simulink model "SimulinkModel"  (R2023b)
settings: Solver=FixedStepAuto  StartTime=0.0  StopTime=10.0  FixedStep=param.rateTransition_Main  RelTol=1e-3  EnableMultiTasking=on
undefined symbols (not defined in the file or in its folder): lidarMeasurement, param, SensorDataOS2, timestamp
libraries: simulink x30, GenericTarget x11, etargetslib x8
(part 2 of 3)

== system SimulinkModel/Send Dynamic Mapping/staticVoxelOccupancyColors ==
  note: uint8 	0x53 bzw 'S'
      | double 	Timestamp
      | uint8  	MaxSegment
      | uint8 	SegmentImdex
      | double 	North East Down Roll Pitch Yaw
      | uint32	FrameID
      | uint32 	num Points
      | uint32	Points : XYZ
      | total 67 bytes
  timestamp : Inport
  pose : Inport  Port=2
  point : Inport  Port=3
  numpoint : Inport  Port=4
  nummsg : Inport  Port=5
  frameID : Inport  Port=6
  Byte Pack1 : etargetslib/Byte Pack  datatypes={'uint8','double','uint8', 'uint8', 'double', 'uint32', 'uint32', 'single'}  byteAlign=1
  Cast To Double1 : DataTypeConversion  OutDataTypeStr=uint8  SaturateOnIntegerOverflow=off  RndMeth=Floor
  Cast To Double2 : DataTypeConversion  OutDataTypeStr=uint8  SaturateOnIntegerOverflow=off  RndMeth=Floor
  Constant1 : Constant  Value=-1  OutDataTypeStr=int32
  Constant2 : Constant  Value=[0x53]  OutDataTypeStr=uint8
  Constant3 : Constant  Value=[0,0,0,0]  OutDataTypeStr=uint8
  Constant4 : Constant  Value=43  OutDataTypeStr=uint32
  Constant5 : Constant  Value=115  OutDataTypeStr=uint32
  Constant6 : Constant  Value=-1  OutDataTypeStr=int32
  Constant7 : Constant  Value=1111  OutDataTypeStr=uint16
  Equal1 : RelationalOperator  Operator===  OutDataTypeStr=boolean  RndMeth=Simplest  InputSameDT=off
  For Iterator : ForIterator  ResetStates=reset  IterationSource=external
  Gain : Gain  Gain=115  OutDataTypeStr=int32
  Gain1 : Gain  Gain=12  OutDataTypeStr=uint32  LockScale=on
  Selector : Selector  NumberOfDimensions=2  IndexMode=Zero-based  InputPortWidth=3  IndexOptions=Select all,Starting index (port)  Indices=[1 3],1  OutputSizes=4e3,115
  Sum : Sum  Inputs=|++
  Sum1 : Sum  Inputs=|++  OutDataTypeStr=uint32
  Sum2 : Sum  Inputs=|++
  Sum3 : Sum  Inputs=|+-
  Switch : Switch  Criteria=u2 > Threshold  SaturateOnIntegerOverflow=off  InputSameDT=off
  UDP Send : GenericTarget/Interface/UDP Send  showDetails=off  interfacePort=1111  interfaceIP=[0,0,0,0]  deviceName=''  prioritySocket=6  allowBroadcast=off  SampleTime=-1
      settings: SourceProductName=Generic Target
  wires:
  Constant2/1 -> Byte Pack1/1
  timestamp/1 -> Byte Pack1/2
  Constant1/1 -> Sum/1
  For Iterator/1 -> Equal1/2, Sum/2
  Sum/1 -> Cast To Double2/1, Gain/1
  numpoint/1 -> Sum3/1
  Gain/1 -> Sum3/2, Selector/2
  point/1 -> Selector/1
  nummsg/1 -> Sum2/1, Equal1/1, For Iterator/1
  Equal1/1 -> Switch/2
  Sum3/1 -> Switch/1
  Constant5/1 -> Switch/3
  Selector/1 -> Byte Pack1/8
  Switch/1 -> Gain1/1, Byte Pack1/7
  frameID/1 -> Byte Pack1/6
  pose/1 -> Byte Pack1/5
  Cast To Double2/1 -> Byte Pack1/4
  Cast To Double1/1 -> Byte Pack1/3
  Sum2/1 -> Cast To Double1/1
  Constant6/1 -> Sum2/2
  Constant4/1 -> Sum1/1
  Gain1/1 -> Sum1/2
  Sum1/1 -> UDP Send/4
  Byte Pack1/1 -> UDP Send/3
  Constant7/1 -> UDP Send/2
  Constant3/1 -> UDP Send/1

== system SimulinkModel/Send Dynamic Mapping/staticVoxelReflectivityColors ==
  note: uint8 	0x53 bzw 'S'
      | double 	Timestamp
      | uint8  	MaxSegment
      | uint8 	SegmentImdex
      | double 	North East Down
      | uint32	FrameID
      | uint32 	num Points
      | uint32	Points : XYZ
      | total 43 bytes
  timestamp : Inport
  pose : Inport  Port=2
  point : Inport  Port=3
  numpoint : Inport  Port=4
  nummsg : Inport  Port=5
  frameID : Inport  Port=6
  Byte Pack1 : etargetslib/Byte Pack  datatypes={'uint8','double','uint8', 'uint8', 'double', 'uint32', 'uint32', 'single'}  byteAlign=1
  Cast To Double1 : DataTypeConversion  OutDataTypeStr=uint8  SaturateOnIntegerOverflow=off  RndMeth=Floor
  Cast To Double2 : DataTypeConversion  OutDataTypeStr=uint8  SaturateOnIntegerOverflow=off  RndMeth=Floor
  Constant1 : Constant  Value=-1  OutDataTypeStr=int32
  Constant2 : Constant  Value=[0x53]  OutDataTypeStr=uint8
  Constant3 : Constant  Value=[0,0,0,0]  OutDataTypeStr=uint8
  Constant4 : Constant  Value=43  OutDataTypeStr=uint32
  Constant5 : Constant  Value=115  OutDataTypeStr=uint32
  Constant6 : Constant  Value=-1  OutDataTypeStr=int32
  Constant7 : Constant  Value=1111  OutDataTypeStr=uint16
  Equal1 : RelationalOperator  Operator===  OutDataTypeStr=boolean  RndMeth=Simplest  InputSameDT=off
  For Iterator : ForIterator  ResetStates=reset  IterationSource=external
  Gain : Gain  Gain=115  OutDataTypeStr=int32
  Gain1 : Gain  Gain=12  OutDataTypeStr=uint32  LockScale=on
  Selector : Selector  NumberOfDimensions=2  IndexMode=Zero-based  InputPortWidth=3  IndexOptions=Select all,Starting index (port)  Indices=[1 3],1  OutputSizes=4e3,115
  Sum : Sum  Inputs=|++
  Sum1 : Sum  Inputs=|++  OutDataTypeStr=uint32
  Sum2 : Sum  Inputs=|++
  Sum3 : Sum  Inputs=|+-
  Switch : Switch  Criteria=u2 > Threshold  SaturateOnIntegerOverflow=off  InputSameDT=off
  UDP Send : GenericTarget/Interface/UDP Send  showDetails=off  interfacePort=1111  interfaceIP=[0,0,0,0]  deviceName=''  prioritySocket=6  allowBroadcast=off  SampleTime=-1
      settings: SourceProductName=Generic Target
  wires:
  Constant2/1 -> Byte Pack1/1
  timestamp/1 -> Byte Pack1/2
  Constant1/1 -> Sum/1
  For Iterator/1 -> Equal1/2, Sum/2
  Sum/1 -> Cast To Double2/1, Gain/1
  numpoint/1 -> Sum3/1
  Gain/1 -> Sum3/2, Selector/2
  point/1 -> Selector/1
  nummsg/1 -> Sum2/1, Equal1/1, For Iterator/1
  Equal1/1 -> Switch/2
  Sum3/1 -> Switch/1
  Constant5/1 -> Switch/3
  Selector/1 -> Byte Pack1/8
  Switch/1 -> Gain1/1, Byte Pack1/7
  frameID/1 -> Byte Pack1/6
  pose/1 -> Byte Pack1/5
  Cast To Double2/1 -> Byte Pack1/4
  Cast To Double1/1 -> Byte Pack1/3
  Sum2/1 -> Cast To Double1/1
  Constant6/1 -> Sum2/2
  Constant4/1 -> Sum1/1
  Gain1/1 -> Sum1/2
  Sum1/1 -> UDP Send/4
  Byte Pack1/1 -> UDP Send/3
  Constant7/1 -> UDP Send/2
  Constant3/1 -> UDP Send/1

== system SimulinkModel/Lidar Message/Lidar:decode/Subsystem ==
  bytes : Inport
  Enable : EnablePort
  Constant11 : Constant  Value=sensorData.n_mm
  Data Store r_min : DataStoreMemory  DataStoreName=r_min  ReadBeforeWriteMsg=warning  WriteAfterWriteMsg=warning  WriteAfterReadMsg=warning  InitialValue=sensorData.r_min-sensorData.n_mm  ShareAcrossModelInstances=on  ShowAdditionalParam=off  OutDataTypeStr=double
  Data Store x_1 : DataStoreMemory  DataStoreName=x_1  ReadBeforeWriteMsg=warning  WriteAfterWriteMsg=warning  WriteAfterReadMsg=warning  InitialValue=sensorData.x_1  ShareAcrossModelInstances=on  ShowAdditionalParam=off  OutDataTypeStr=double
  Data Store x_2 : DataStoreMemory  DataStoreName=x_2  ReadBeforeWriteMsg=warning  WriteAfterWriteMsg=warning  WriteAfterReadMsg=warning  InitialValue=sensorData.x_2  ShareAcrossModelInstances=on  ShowAdditionalParam=off  OutDataTypeStr=double
  Data Store y_1 : DataStoreMemory  DataStoreName=y_1  ReadBeforeWriteMsg=warning  WriteAfterWriteMsg=warning  WriteAfterReadMsg=warning  InitialValue=sensorData.y_1  ShareAcrossModelInstances=on  ShowAdditionalParam=off  OutDataTypeStr=double
  Data Store y_2 : DataStoreMemory  DataStoreName=y_2  ReadBeforeWriteMsg=warning  WriteAfterWriteMsg=warning  WriteAfterReadMsg=warning  InitialValue=sensorData.y_2  ShareAcrossModelInstances=on  ShowAdditionalParam=off  OutDataTypeStr=double
  Data Store z_1 : DataStoreMemory  DataStoreName=z_1  ReadBeforeWriteMsg=warning  WriteAfterWriteMsg=warning  WriteAfterReadMsg=warning  InitialValue=sensorData.z_1  ShareAcrossModelInstances=on  ShowAdditionalParam=off  OutDataTypeStr=double
  Data Store z_2 : DataStoreMemory  DataStoreName=z_2  ReadBeforeWriteMsg=warning  WriteAfterWriteMsg=warning  WriteAfterReadMsg=warning  InitialValue=sensorData.z_2  ShareAcrossModelInstances=on  ShowAdditionalParam=off  OutDataTypeStr=double
  LIDAR:measurement : MATLAB Function  TreatAsAtomicUnit=on
  wires:
  Constant11/1 -> LIDAR:measurement/2(n_mm)
  bytes/1 -> LIDAR:measurement/1(bytes)

== system SimulinkModel/Lidar Message/SendLidar/Subsystem ==
  In1 : Inport
  Enable : EnablePort
  Out1 : Outport
  wires:
  In1/1 -> Out1/1

== system SimulinkModel/Lidar Message/SendLidar/deltaUnixUtc ==
  Constant : Constant  Value=-1690934400
  Signal Specification31 : SignalSpecification  OutDataTypeStr=double  Unit=s  Dimensions=1
  Sum2 : Sum  Commented=on  Inputs=|-+
  UNIX Time2 : GenericTarget/Time/UNIX Time  Commented=on  SampleTime=-1
      settings: SourceProductName=Generic Target
  UTC Timestamp2 : GenericTarget/Time/UTC Timestamp  Commented=on  SampleTime=-1
      settings: SourceProductName=Generic Target
  deltaUnixUtc : Outport
  wires:
  Constant/1 -> Signal Specification31/1
  Signal Specification31/1 -> deltaUnixUtc/1  "reset"
  UTC Timestamp2/1 -> Sum2/2
  UNIX Time2/1 -> Sum2/1

== system SimulinkModel/Navigation Message/NavMsg/Subsystem ==
  Bytes : Inport
  Length : Inport  Port=2
  timestampGT : Inport  Port=3
  Enable : EnablePort
  Detect Change : simulink/Logic and Bit Operations/Detect Change  vinit=0  OutDataTypeStr=boolean
  Subsystem : Subsystem
  UDP Interface In Host : Subsystem
  measurement : Outport
  wires:
  Bytes/1 -> UDP Interface In Host/1(Bytes)
  Length/1 -> UDP Interface In Host/2(Length)
  Subsystem/1(measurementOut) -> measurement/1
  Detect Change/1 -> Subsystem/Enable
  timestampGT/1 -> UDP Interface In Host/3(timestampGT), Detect Change/1
  UDP Interface In Host/1(BelaPosVelBus) -> Subsystem/1(measurement)

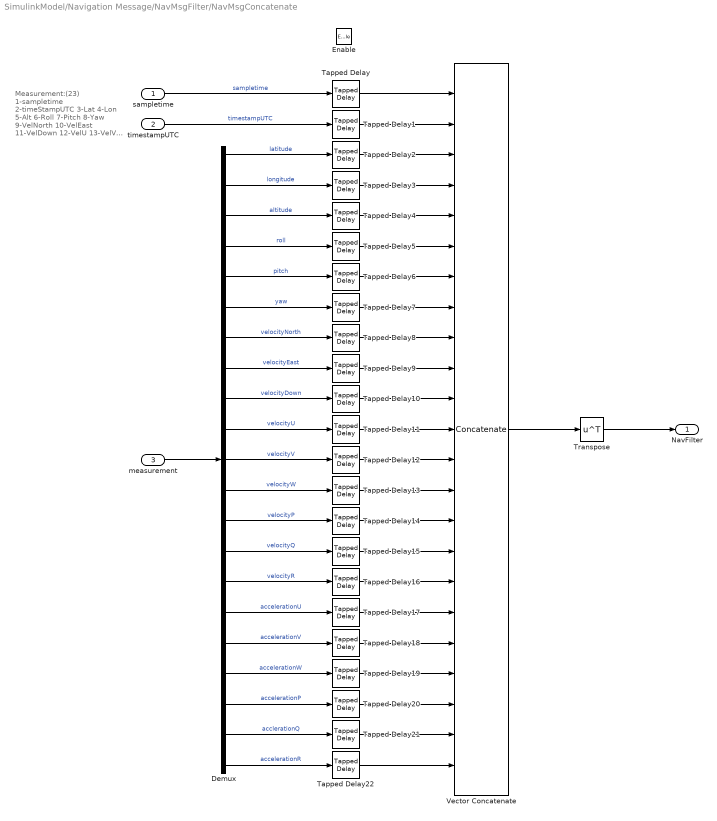
== system SimulinkModel/Navigation Message/NavMsgFilter/NavMsgConcatenate ==
  note: Measurement:(23)
      | 	1-sampletime
      | 	2-timeStampUTC
      | 	3-Lat
      | 	4-Lon
      | 	5-Alt
      | 	6-Roll
      | 	7-Pitch
      | 	8-Yaw
      | 	9-VelNorth
      | 	10-VelEast
      | 	11-VelDown
      | 	12-VelU
      | 	13-VelV
      | 	14-VelW
      | 	15-VelP
      | 	16-VelQ
      | 	17-VelR
      | 	18-AccU
      | 	19-AccV
      | 	20-AccW
      | 	21-AccP
      | 	22-AccQ
      | 	23-AccR
  sampletime : Inport
  timestampUTC : Inport  Port=2
  measurement : Inport  Port=3
  Enable : EnablePort
  Demux : Demux  Outputs=21
  Tapped Delay{,1..22} (23 alike) : simulink/Discrete/Tapped Delay  vinit=0.0  samptime=-1  NumDelays=numDelay  DelayOrder=Oldest  includeCurrent=off
  Transpose : Math  Operator=transpose
  Vector Concatenate : Concatenate  NumInputs=23  Mode=Multidimensional array  ConcatenateDimension=2
  NavFilter : Outport
  wires:
  sampletime/1 -> Tapped Delay/1  "sampletime"
  measurement/1 -> Demux/1
  timestampUTC/1 -> Tapped Delay1/1  "timestampUTC"
  Demux/1 -> Tapped Delay2/1  "latitude"
  Demux/2 -> Tapped Delay3/1  "longitude"
  Demux/3 -> Tapped Delay4/1  "altitude"
  Demux/4 -> Tapped Delay5/1  "roll"
  Demux/5 -> Tapped Delay6/1  "pitch"
  Demux/6 -> Tapped Delay7/1  "yaw"
  Demux/7 -> Tapped Delay8/1  "velocityNorth"
  Demux/8 -> Tapped Delay9/1  "velocityEast"
  Demux/9 -> Tapped Delay10/1  "velocityDown"
  Demux/10 -> Tapped Delay11/1  "velocityU"
  Demux/11 -> Tapped Delay12/1  "velocityV"
  Demux/12 -> Tapped Delay13/1  "velocityW"
  Demux/13 -> Tapped Delay14/1  "velocityP"
  Demux/14 -> Tapped Delay15/1  "velocityQ"
  Demux/15 -> Tapped Delay16/1  "velocityR"
  Demux/16 -> Tapped Delay17/1  "accelerationU"
  Demux/17 -> Tapped Delay18/1  "accelerationV"
  Demux/18 -> Tapped Delay19/1  "accelerationW"
  Demux/19 -> Tapped Delay20/1  "accelerationP"
  Demux/20 -> Tapped Delay21/1  "acclerationQ"
  Demux/21 -> Tapped Delay22/1  "accelerationR"
  Tapped Delay/1 -> Vector Concatenate/1
  Tapped Delay1/1 -> Vector Concatenate/2
  Tapped Delay2/1 -> Vector Concatenate/3
  Tapped Delay3/1 -> Vector Concatenate/4
  Tapped Delay4/1 -> Vector Concatenate/5
  Tapped Delay5/1 -> Vector Concatenate/6
  Tapped Delay6/1 -> Vector Concatenate/7
  Tapped Delay7/1 -> Vector Concatenate/8
  Tapped Delay8/1 -> Vector Concatenate/9
  Tapped Delay9/1 -> Vector Concatenate/10
  Tapped Delay10/1 -> Vector Concatenate/11
  Tapped Delay12/1 -> Vector Concatenate/13
  Tapped Delay11/1 -> Vector Concatenate/12
  Tapped Delay13/1 -> Vector Concatenate/14
  Tapped Delay14/1 -> Vector Concatenate/15
  Tapped Delay15/1 -> Vector Concatenate/16
  Tapped Delay16/1 -> Vector Concatenate/17
  Tapped Delay17/1 -> Vector Concatenate/18
  Tapped Delay18/1 -> Vector Concatenate/19
  Tapped Delay19/1 -> Vector Concatenate/20
  Tapped Delay20/1 -> Vector Concatenate/21
  Tapped Delay21/1 -> Vector Concatenate/22
  Tapped Delay22/1 -> Vector Concatenate/23
  Vector Concatenate/1 -> Transpose/1
  Transpose/1 -> NavFilter/1

== system SimulinkModel/Processing Data/ProcessData/ProcessData ==
  Lidar : Inport
  Enable : EnablePort
  processData : MATLAB Function  TreatAsAtomicUnit=on
  Lidar_ : Outport
  wires:
  Lidar/1 -> processData/1(Lidar)
  processData/1(Lidar_) -> Lidar_/1

== system SimulinkModel/Navigation Message/NavMsg/Subsystem/Subsystem ==
  measurement : Inport
  Enable : EnablePort
  measurementOut : Outport
  wires:
  measurement/1 -> measurementOut/1

== system SimulinkModel/Navigation Message/NavMsg/Subsystem/UDP Interface In Host ==
  Bytes : Inport  OutDataTypeStr=uint8
  Length : Inport  Port=2
  timestampGT : Inport  Port=3
  Decode Bytes : Subsystem
  BelaPosVelBus : Outport
  wires:
  Bytes/1 -> Decode Bytes/1(Bytes)
  Length/1 -> Decode Bytes/Enable
  Decode Bytes/1(BelaPosVelBus) -> BelaPosVelBus/1
  timestampGT/1 -> Decode Bytes/2(timestampGT)

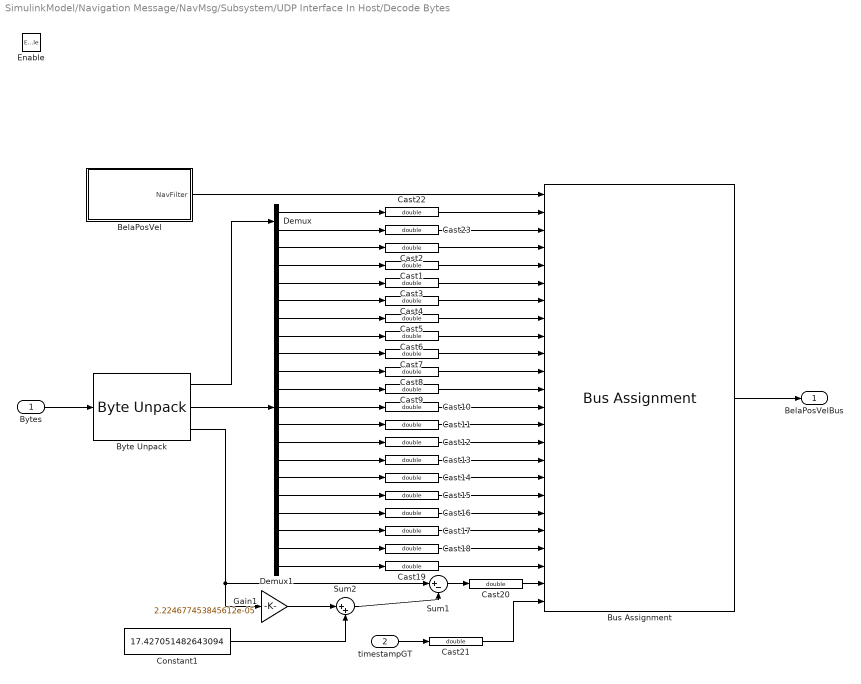
== system SimulinkModel/Navigation Message/NavMsg/Subsystem/UDP Interface In Host/Decode Bytes ==
  Bytes : Inport
  timestampGT : Inport  Port=2
  Enable : EnablePort
  BelaPosVel : Subsystem
  Bus Assignment : BusAssignment  AssignedSignals=measurement.latitude,measurement.longitude,measurement.altitude,measurement.roll,measurement.pitch,measurement.yaw,measurement.velocityU,measurement.velocityV,measurement.velocityW,measurement.velocityP,measurement.velocityQ,measurement.velocityR,measurement.accelerationU,measurement.accelerationV,measurement.accelerationW,measurement.accelerationP,measurement.accelerationQ,measurement.accelerationR,measurement.velocityNorth,measurement.velocityEast,measurement.velocityDown,timestamp.timestampUTC,timestamp.timestampGT
  Byte Unpack : etargetslib/Byte Unpack  dimensions={2,19,1}  datatypes={'double','single','double'}  byteAlign=1
  Cast{1..23} (23 alike) : DataTypeConversion  OutDataTypeStr=double  SaturateOnIntegerOverflow=off  RndMeth=Floor
  Constant1 : Constant  Value=17.427051482643094
  Demux : Demux  Outputs=2
  Demux1 : Demux  Outputs=19
  Gain1 : Gain  Gain=2.224677453845612e-05
  Sum1 : Sum  Inputs=|+-
  Sum2 : Sum  Inputs=|++
  BelaPosVelBus : Outport
  wires:
  Bytes/1 -> Byte Unpack/1
  Byte Unpack/1 -> Demux/1
  Byte Unpack/2 -> Demux1/1
  Bus Assignment/1 -> BelaPosVelBus/1
  Constant1/1 -> Sum2/2
  Gain1/1 -> Sum2/1
  Sum2/1 -> Sum1/2
  Byte Unpack/3 -> Sum1/1, Gain1/1
  Sum1/1 -> Cast20/1
  timestampGT/1 -> Cast21/1
  Demux/1 -> Cast22/1
  Demux/2 -> Cast23/1
  Demux1/1 -> Cast2/1
  Demux1/2 -> Cast1/1
  Demux1/3 -> Cast3/1
  Demux1/4 -> Cast4/1
  Demux1/5 -> Cast5/1
  Demux1/6 -> Cast6/1
  Demux1/7 -> Cast7/1
  Demux1/8 -> Cast8/1
  Demux1/9 -> Cast9/1
  Demux1/10 -> Cast10/1
  Demux1/11 -> Cast11/1
  Demux1/12 -> Cast12/1
  Demux1/13 -> Cast13/1
  Demux1/14 -> Cast14/1
  Demux1/15 -> Cast15/1
  Demux1/16 -> Cast16/1
  Demux1/17 -> Cast17/1
  Demux1/18 -> Cast18/1
  Demux1/19 -> Cast19/1
  Cast2/1 -> Bus Assignment/4
  Cast1/1 -> Bus Assignment/5
  Cast3/1 -> Bus Assignment/6
  Cast4/1 -> Bus Assignment/7
  Cast5/1 -> Bus Assignment/8
  Cast6/1 -> Bus Assignment/9
  Cast7/1 -> Bus Assignment/10
  Cast8/1 -> Bus Assignment/11
  Cast9/1 -> Bus Assignment/12
  Cast10/1 -> Bus Assignment/13
  Cast11/1 -> Bus Assignment/14
  Cast12/1 -> Bus Assignment/15
  Cast13/1 -> Bus Assignment/16
  Cast14/1 -> Bus Assignment/17
  Cast15/1 -> Bus Assignment/18
  Cast16/1 -> Bus Assignment/19
  Cast17/1 -> Bus Assignment/20
  Cast18/1 -> Bus Assignment/21
  Cast19/1 -> Bus Assignment/22
  Cast22/1 -> Bus Assignment/2
  Cast23/1 -> Bus Assignment/3
  BelaPosVel/1(NavFilter) -> Bus Assignment/1
  Cast20/1 -> Bus Assignment/23
  Cast21/1 -> Bus Assignment/24

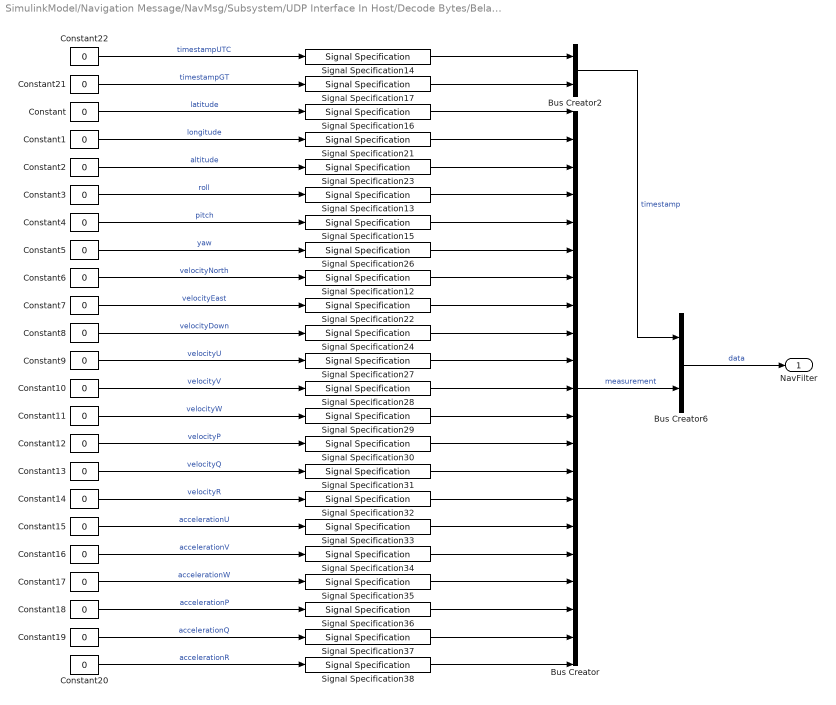
== system SimulinkModel/Navigation Message/NavMsg/Subsystem/UDP Interface In Host/Decode Bytes/BelaPosVel ==
  Bus Creator : BusCreator  Inputs=21
  Bus Creator2 : BusCreator  Inputs=2
  Bus Creator6 : BusCreator  Inputs=2
  Constant{,1..22} (23 alike) : Constant  Value=0  OutDataTypeStr=double
  Signal Specification{12,22,24,27..29} (6 alike) : SignalSpecification  OutDataTypeStr=double  Unit=m/s  Dimensions=1
  Signal Specification{13,15..16,21,23,26} (6 alike) : SignalSpecification  OutDataTypeStr=double  Unit=rad  Dimensions=1
  Signal Specification14 : SignalSpecification  OutDataTypeStr=double  Unit=s  Dimensions=1
  Signal Specification17 : SignalSpecification  OutDataTypeStr=double  Unit=s  Dimensions=1
  Signal Specification30 : SignalSpecification  OutDataTypeStr=double  Unit=rad/s  Dimensions=1
  Signal Specification31 : SignalSpecification  OutDataTypeStr=double  Unit=rad/s  Dimensions=1
  Signal Specification32 : SignalSpecification  OutDataTypeStr=double  Unit=rad/s  Dimensions=1
  Signal Specification33 : SignalSpecification  OutDataTypeStr=double  Unit=m/s^2  Dimensions=1
  Signal Specification34 : SignalSpecification  OutDataTypeStr=double  Unit=m/s^2  Dimensions=1
  Signal Specification35 : SignalSpecification  OutDataTypeStr=double  Unit=m/s^2  Dimensions=1
  Signal Specification36 : SignalSpecification  OutDataTypeStr=double  Unit=rad/s^2  Dimensions=1
  Signal Specification37 : SignalSpecification  OutDataTypeStr=double  Unit=rad/s^2  Dimensions=1
  Signal Specification38 : SignalSpecification  OutDataTypeStr=double  Unit=rad/s^2  Dimensions=1
  NavFilter : Outport
  wires:
  Constant21/1 -> Signal Specification17/1  "timestampGT"
  Constant2/1 -> Signal Specification23/1  "altitude"
  Constant5/1 -> Signal Specification26/1  "yaw"
  Constant20/1 -> Signal Specification38/1  "accelerationR"
  Constant1/1 -> Signal Specification21/1  "longitude"
  Constant4/1 -> Signal Specification15/1  "pitch"
  Constant6/1 -> Signal Specification12/1  "velocityNorth"
  Constant7/1 -> Signal Specification22/1  "velocityEast"
  Constant/1 -> Signal Specification16/1  "latitude"
  Constant3/1 -> Signal Specification13/1  "roll"
  Constant8/1 -> Signal Specification24/1  "velocityDown"
  Constant16/1 -> Signal Specification34/1  "accelerationV"
  Constant13/1 -> Signal Specification31/1  "velocityQ"
  Constant9/1 -> Signal Specification27/1  "velocityU"
  Constant12/1 -> Signal Specification30/1  "velocityP"
  Constant11/1 -> Signal Specification29/1  "velocityW"
  Constant10/1 -> Signal Specification28/1  "velocityV"
  Constant17/1 -> Signal Specification35/1  "accelerationW"
  Constant14/1 -> Signal Specification32/1  "velocityR"
  Constant15/1 -> Signal Specification33/1  "accelerationU"
  Constant18/1 -> Signal Specification36/1  "accelerationP"
  Constant19/1 -> Signal Specification37/1  "accelerationQ"
  Constant22/1 -> Signal Specification14/1  "timestampUTC"
  Bus Creator6/1 -> NavFilter/1  "data"
  Bus Creator2/1 -> Bus Creator6/1  "timestamp"
  Signal Specification14/1 -> Bus Creator2/1
  Signal Specification17/1 -> Bus Creator2/2
  Bus Creator/1 -> Bus Creator6/2  "measurement"
  Signal Specification16/1 -> Bus Creator/1
  Signal Specification21/1 -> Bus Creator/2
  Signal Specification23/1 -> Bus Creator/3
  Signal Specification13/1 -> Bus Creator/4
  Signal Specification15/1 -> Bus Creator/5
  Signal Specification26/1 -> Bus Creator/6
  Signal Specification12/1 -> Bus Creator/7
  Signal Specification22/1 -> Bus Creator/8
  Signal Specification24/1 -> Bus Creator/9
  Signal Specification27/1 -> Bus Creator/10
  Signal Specification28/1 -> Bus Creator/11
  Signal Specification29/1 -> Bus Creator/12
  Signal Specification30/1 -> Bus Creator/13
  Signal Specification31/1 -> Bus Creator/14
  Signal Specification32/1 -> Bus Creator/15
  Signal Specification33/1 -> Bus Creator/16
  Signal Specification34/1 -> Bus Creator/17
  Signal Specification35/1 -> Bus Creator/18
  Signal Specification36/1 -> Bus Creator/19
  Signal Specification37/1 -> Bus Creator/20
  Signal Specification38/1 -> Bus Creator/21

== matlab function SimulinkModel/Processing Data/ProcessData/ProcessData/processData ==
  data: Lidar input Bus: busRawSensorMessage_LidarOdometry; Lidar_ output Bus: busRawSensorMessage_LidarOdometry
function Lidar_  = processData(Lidar)

    numberPoints = Lidar.lidarMeasurement.numberPoint;
    points = Lidar.lidarMeasurement.points;
    pointReflect = Lidar.lidarMeasurement.pointsReflect;
    pointTimestamps = Lidar.lidarMeasurement.pointsTimestamp;
    pointsMeasurementIDs = Lidar.lidarMeasurement.pointsMeasurementID;

    [numberPoints_,points_,pointReflect_,pointTimestamps_,pointsMeasurementIDs_,~] = downsample(numberPoints,points,pointReflect,pointTimestamps,pointsMeasurementIDs);

    Lidar_ = Lidar;
    Lidar_.lidarMeasurement2.numberPoint = numberPoints_;
    Lidar_.lidarMeasurement2.points = points_;
    Lidar_.lidarMeasurement2.pointsReflect = pointReflect_;
    Lidar_.lidarMeasurement2.pointsTimestamp = pointTimestamps_;
    Lidar_.lidarMeasurement2.pointsMeasurementID = pointsMeasurementIDs_;
    
end


function [numberPoints_,points_,pointReflect_,pointTimestamps_,pointsMeasurementIDs_,vs_] = downsample(numberPoints,points,pointReflect,pointTimestamps,pointsMeasurementIDs)

    fixNumberPoints = 128*1024;

    minDist = 10;
    maxDist = 200;

    pointsBody = points(1:numberPoints,1:3);
    pointReflectBody = pointReflect(1:numberPoints,1:3);
    pointTimestampsBody = pointTimestamps(1:numberPoints,1);
    pointsMeasurementIDsBody = pointsMeasurementIDs(1:numberPoints,1);

    points_ = NaN(fixNumberPoints,3,'single');
    pointReflect_ = NaN(fixNumberPoints,3,'single');
    pointTimestamps_ = NaN(fixNumberPoints,1,'double');
    pointsMeasurementIDs_ = NaN(fixNumberPoints,1,'single');

    x = pointsBody(:,1);
    y = pointsBody(:,2);
    z = pointsBody(:,3);

    vs1 = 1;
    % vs2 = 1.5;

    vx1 = floor(x*(1/vs1));
    vy1 = floor(y*(1/vs1));
    vz1 = floor(z*(1/vs1));

    % vx2 = floor(x*(1/vs2));
    % vy2 = floor(y*(1/vs2));
    % vz2 = floor(z*(1/vs2));

    struct1 = [x y z vx1 vy1 vz1 pointReflectBody pointTimestampsBody pointsMeasurementIDsBody];
    % struct2 = [x y z vx2 vy2 vz2 pointReflectBody pointTimestampsBody pointsMeasurementIDsBody];

    [~,ia1] = unique(struct1(1:numberPoints,4:6),"rows");
    % [~,ia2] = unique(struct2(1:numberPoints,4:6),"rows");

    %updatedStruct = struct1(ia1,:);
   

    updatedStruct1 = struct1(ia1,:);
    % updatedStruct2 = struct2(ia2,:);

    % height1 = height(updatedStruct1);
    % height2 = height(updatedStruct2);

    % height0 = [height1 height2];

    % [~,idx] = mink(abs(height0(1,:) - 8000),2);

    %search for first downsample
    % if idx(1) == 1
    %     updatedStruct = updatedStruct1;
    %     vs_ = vs1;
    % else
    %     updatedStruct = updatedStruct2;
    %     vs_ = vs2;
    % end

    updatedStruct = updatedStruct1;
    vs_ = vs1;

    pointDist = sqrt(sum((updatedStruct(:,1:3)).^2,2));
    ib = pointDist > minDist & pointDist < maxDist;
    updatedUpdatedStruct = updatedStruct(ib,:);

    numP = height(updatedUpdatedStruct);

    %vs_ = vs1;

    points_(1:numP,1:3) =  single(updatedUpdatedStruct(1:numP,1:3));
    pointReflect_(1:numP,1:3) = single(updatedUpdatedStruct(1:numP,7:9));
    pointTimestamps_(1:numP,1) = double(updatedUpdatedStruct(1:numP,10));
    pointsMeasurementIDs_(1:numP,1) = single(updatedUpdatedStruct(1:numP,11));
    numberPoints_ = uint32(numP);

end

== matlab function SimulinkModel/Lidar Message/Lidar:decode/Subsystem/LIDAR:measurement ==
  data: bytes input uint8 size=24896; n_mm input; x_1 data_store_memory; x_2 data_store_memory; y_1 data_store_memory; y_2 data_store_memory; z_1 data_store_memory; r_min data_store_memory; Cnt_1v2 data_store_memory; Speicher_1v2 data_store_memory; z_2 data_store_memory; Speicher1_numPoints_body data_store_memory; Speicher1_XYZ_body data_store_memory; Speicher1_M_ID_body data_store_memory; Speicher1_timestamp_body data_store_memory; Speicher1_Reflect_body data_store_memory
function lidarMeasurement(bytes,n_mm)

global x_1
global x_2
global y_1
global y_2
global z_1
global z_2
global r_min
global Cnt_1v2;
global Speicher_1v2;

%##############################################

global Speicher1_numPoints_body;
global Speicher1_XYZ_body;
global Speicher1_M_ID_body;
global Speicher1_timestamp_body;
global Speicher1_Reflect_body;

%##############################################

persistent frame_id;
persistent decoded_blocks;

if isempty(frame_id)
   frame_id = uint16(0);
   decoded_blocks = 0; 
end
% 1) take the last measurement block's time as message time.
% 23340 = 1556*15 bytes
%temp = typecast(bytes(23340+(1:8)), 'uint64'); % get the 16th block time message
%timestamp0 = double(temp)*1e-9;                % initialize

for block = 0:2:15 % 0:2:15 for 2048 resolution % 0:15 for 1024 resolution
    offset_block = block * 1556 + 1;                                            % bytes offset of each block % 1556 bytes per Block % NOTE: measurement block
    temp = typecast(bytes(offset_block+(0:7)), 'uint64');                       % get the respective block time
    timestamp = double(temp)*1e-9;                                              % timestamp each block in second
    M_ID = typecast(bytes(offset_block+(8:9)), 'uint16') + uint16(1);           % measurement ID
    F_ID = typecast(bytes(offset_block+(10:11)), 'uint16') + uint16(1);         % frame ID

    %% ####################################
    if F_ID ~= frame_id                                                         % start new frame ID
        frame_id = F_ID;
         if decoded_blocks == 1024                                             % decode block is for counter trigger
            if Speicher_1v2 == uint8(1)
                Speicher_1v2 = uint8(2);
                Cnt_1v2 = uint8(1);
                Speicher1_numPoints_body(1) = uint32(0);
            else
                Speicher_1v2 = uint8(1);
                Cnt_1v2 = uint8(2);
                Speicher1_numPoints_body(2) = uint32(0);
            end
         else
                Speicher1_numPoints_body(Cnt_1v2) = uint32(0);
         end
          decoded_blocks = 0;
    end
    %% ####################################
    cnt = Cnt_1v2;                                                              % speicher bereich
    numP_body = Speicher1_numPoints_body(cnt);                                  % declare num body set

    if isequal(bytes(offset_block+(1552:1555)) , [0xFF 0xFF 0xFF 0xFF]')        % if measurement block status is valid
        offset_block = offset_block + 4;                                        % Header 16 bytes - first Channel (12bytes) % 4 is to skip encoder count
        for channel = 1:2:128                                                     % eval_channel %[1:4:57, 60:2:70, 70:3:128]%
            offset_ch = offset_block + channel*12;
            Range =  double(typecast([bytes(offset_ch+(0:2)); 0x00], 'uint32'))-n_mm;
            if Range > r_min(channel, M_ID)
                XYZ =  [Range*x_1(channel, M_ID)+x_2(M_ID);...                  % berechnen XYZ
                             Range*y_1(channel, M_ID)+y_2(M_ID);...
                             Range*z_1(channel, M_ID)+z_2(M_ID)].*1e-3;
                %###################################################
                %Z = XYZ(3);
                %if Z < 0 
                    numP_body = numP_body +uint32(1);
                    Speicher1_XYZ_body(numP_body, 1:3, cnt) = XYZ';             % IN MM OR IN M
                    Speicher1_M_ID_body(numP_body, cnt) = M_ID;
                    Speicher1_timestamp_body(numP_body, cnt) = timestamp;
                    Speicher1_Reflect_body(numP_body, 1, cnt) =  typecast([bytes(offset_ch+(4)); 0x00], 'uint16');
                    Speicher1_Reflect_body(numP_body, 2, cnt) =  typecast(bytes(offset_ch+(6:7)), 'uint16');
                    Speicher1_Reflect_body(numP_body, 3, cnt) =  typecast(bytes(offset_ch+(8:9)), 'uint16');
                %end
                %###################################################
            end    
        end
       %########################################
       Speicher1_numPoints_body(cnt) = numP_body;
       %########################################

    end
    %% ####################################
    decoded_blocks = decoded_blocks+1;
end

== matlab function SimulinkModel/Dynamic Mapping/MATLAB Function ==
  data: Point input; points_ output; numPoint input; N input; E input; D input; qw input; qx input; qy input; qz input
function points_ = fcn(Point,numPoint,N,E,D,qw,qx,qy,qz)
    
    points_ = NaN(131072,3,'single');
    
    p = Point(1:numPoint,:);
    
    currOdom = [N,E,D,qw,qx,qy,qz];
    T = TransformMatrix(currOdom);
    Pout = PointTransform(p,T);
    points_(1:np,:) = Pout;
end



function Pout = PointTransform(Point,T)
    Pout = Point * T(1:3,1:3)';
    Pout(:,1) = Pout(:,1) +T(1,4);
    Pout(:,2) = Pout(:,2) +T(2,4);
    Pout(:,3) = Pout(:,3) +T(3,4);
end

function T = TransformMatrix(x)
    q = x(4:7);
    q = (reshape(q,1,4))';
    C = Cb2n(q);
    T = eye(4);
    T(1:3,1:3) = C;
    p = x(1:3);
    p = (reshape(p,1,3))';
    T(1:3,4) = p;
end
